simulink model "threephaseinverterwithonetwenty"  (R2013b)
settings: Solver=ode45  StartTime=0.0  StopTime=10.0  RelTol=1e-3
libraries: elec_lib x14, fl_lib x2, powerlib x1
settings Model: Creator=SAI KUMAR  LastModifiedBy=SAI KUMAR

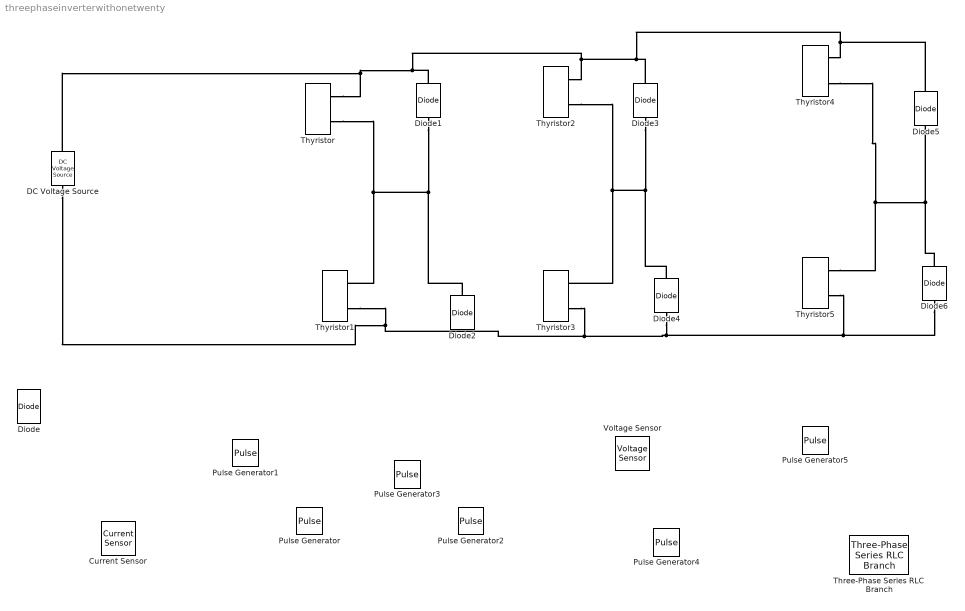
== system threephaseinverterwithonetwenty ==
  Current Sensor : fl_lib/Electrical/Electrical Sensors/Current Sensor  i1_Log=off  v1_Log=off  LocalVarNames=|i1|v1  LocalVarDescs=|i1|v1  LocalVarLogging=[0 0]
  DC Voltage Source : elec_lib/Additional Components/SPICE-Compatible Components/Sources/DC Voltage Source  DC=0 V  i_Log=off  LocalVarNames=|i  LocalVarDescs=|i  LocalVarLogging=0
  Diode{,1..6} (7 alike) : elec_lib/Semiconductor Devices/Diode  ModelType=1  Vf=0.6 V  Ron=0.3 Ohm  Goff=1e-8 S  Rz=0.3 Ohm  Vz=50 V  C_PWL=5 pF  prmExp=1  I12=[ 0.0137 0.545 ] A  V12=[ 0.6 0.7 ] V  I1=0.0137 A  V1=0.6 V  RS=0.01 Ohm  IS=1e-12 A  Tmeas=25 C  ec=1  BV=Inf V  C_param=1  CJ0=5 pF  VJ=1 V  Mgrad=0.5  Vvec=[ 0.1 10 100 ] V  Cvec=[ 3.5 1 0.4 ] pF  FC=0.5  Q_param=1  Irrm=-7.15 A  iF=4 A  didt=-750 A/us  trr=115 ns  TT=50 ns  tau=100 ns  T_param=1  IS_T2=1.25e-7 A  I1_T2=0.245 A  V1_T2=0.5 V  Tmeas2=125 C  EG_param=1  EG=1.11 eV  XTI_param=1  XTI=3  dBVdT=0 V/K  Tdevice=25 C  LocalVarLogging=[]  Rth=[ 0 10 ] K/W  thermal_mass_parameterization=1  thermal_mass=[ 0 1 ] J/K  thermal_time_constant=[ 0 10 ] s  thermal_mass_initial_temperatures=[ 25 25 ] C
  Pulse Generator{,1..5} (6 alike) : DiscretePulseGenerator  PulseType=Time based  Period=10  PulseWidth=5
  Three-Phase Series RLC Branch : powerlib/Elements/Three-Phase Series RLC Branch  LConnTagsString=A|B|C  RConnTagsString=A|B|C  BranchType=R  Resistance=1000  Inductance=1e-3  Capacitance=1e-6  Measurements=None
  Thyristor{,1..5} (6 alike) : elec_lib/Semiconductor Devices/Thyristor  v_on=1.2 V  i_on=1 A  IDRM=0.01 mA  VDRM=400 V  Tmeas=25 C  i_GT=3 uA  v_GT=0.6 V  V_D=12 V  R=120 Ohm  dVdt=150 V/us  R_GK=1000 Ohm  TF_NPN_parameterization=1  T_d=2 us  i_d=10 mA  TF_NPN=0.3 us  TF_PNP_parameterization=1  TF_PNP=0.3 us  Rs=87 kOhm  Rgate=10 Ohm  Gain=10  LocalVarLogging=[]  Rth=[ 0 10 ] K/W  thermal_mass_parameterization=1  thermal_mass=[ 0 1 ] J/K  thermal_time_constant=[ 0 10 ] s  thermal_mass_initial_temperatures=[ 25 25 ] C
  Voltage Sensor : fl_lib/Electrical/Electrical Sensors/Voltage Sensor  i1_Log=off  v1_Log=off  LocalVarNames=|i1|v1  LocalVarDescs=|i1|v1  LocalVarLogging=[0 0]
  connections:
  Thyristor/RConn1 -- DC Voltage Source/LConn1 -- Diode1/RConn1 -- Diode5/RConn1 -- Thyristor4/RConn1 -- Diode3/RConn1 -- Thyristor2/RConn1
  Thyristor3/RConn2 -- Diode6/LConn1 -- Thyristor5/RConn2 -- Diode4/LConn1 -- DC Voltage Source/RConn1 -- Thyristor1/RConn2
  Diode2/RConn1 -- Diode1/LConn1 -- Thyristor1/RConn1 -- Thyristor/RConn2
  Diode4/RConn1 -- Diode3/LConn1 -- Thyristor3/RConn1 -- Thyristor2/RConn2
  Thyristor4/RConn2 -- Thyristor5/RConn1 -- Diode5/LConn1 -- Diode6/RConn1
